simulink model "Inverter_bldc"  (R2020b)
settings: Solver=VariableStepAuto  StartTime=0.0  StopTime=10.0  RelTol=1e-3
undefined symbols (not defined in the file or in its folder): inv
settings Model: Creator=giuli  LastModifiedBy=giuli

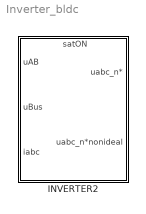
== system Inverter_bldc ==
  INVERTER2 : Subsystem
      settings: PortSchema="{\"entries\":[{\"content\":{\"sides\":[{\"content\":{\"connectorIds\":[\"In1\",\"In2\",\"In3\"]},\"type\":\"ConnectorPlacement.EquallySpacedRectSide\",\"uuid\":\"79c77d12-022f-42ce-98d0-f3ead9d04a95\"},{\"content\":{\"connectorIds\":[\"Out1\",\"Out2\"],\"side\":\"RIGHT\"},\"type\":\"ConnectorPlacement.EquallySpacedRectSide\",\"uuid\":\"afd498dc-a72a-45ee-96a4-44488bf591ce\"},{\"content\":{\"connectorIds\":[\"Out3\"],\"side\":\"TOP\"},\"type\":\"ConnectorPlacement.EquallySpacedRectSide\",\"uuid\":\"f8f8ad46-d0da-4286-941c-855cc15ed51d\"}]},\"type\":\"ConnectorPlacement.EquallySpacedConnector\",\"uuid\":\"436ef73d-4718-409e-82fb-57ff2ccd93cf\"}],\"packageUris\":[\"http://schema.mathworks.com/mf0/Connector/R2020b\"],\"version\":\"1.0\"}"

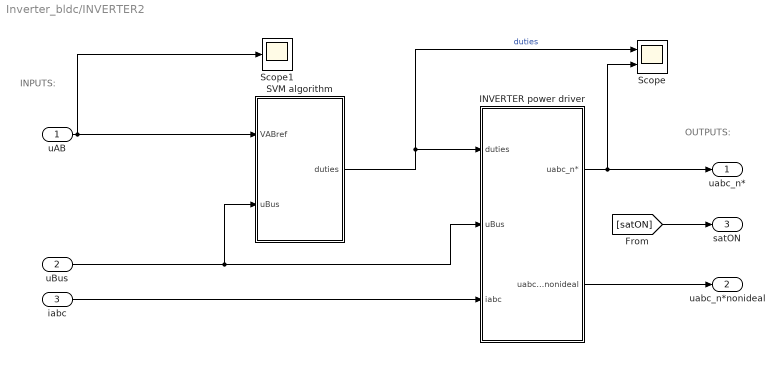
== system Inverter_bldc/INVERTER2 ==
  note: OUTPUTS:
  note: INPUTS:
  uAB : Inport
  uBus : Inport  Port=2
  iabc : Inport  Port=3
  INVERTER power driver : Subsystem
  SVM algorithm : Subsystem
  Scope : Scope  NumInputPorts=2
  Scope1 : Scope
  uabc_n* : Outport
  uabc_n*nonideal : Outport  Port=2
  satON : Outport  Port=3
  wires:
  INVERTER power driver/2(uabc_n*nonideal) -> uabc_n*nonideal/1
  iabc/1 -> INVERTER power driver/3(iabc)
  SVM algorithm/1(duties) -> Scope/1, INVERTER power driver/1(duties)  "duties"
  [satON] -> satON/1
  uBus/1 -> INVERTER power driver/2(uBus), SVM algorithm/2(uBus)
  uAB/1 -> Scope1/1, SVM algorithm/1(VABref)
  INVERTER power driver/1(uabc_n*) -> Scope/2, uabc_n*/1

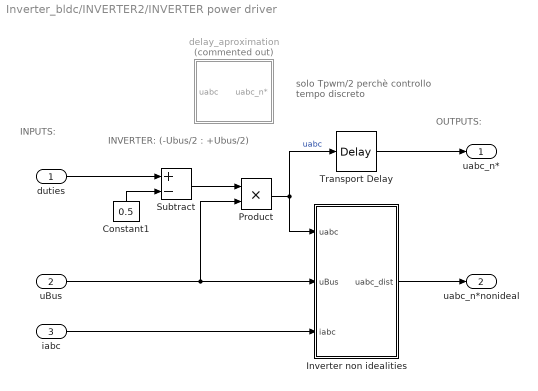
== system Inverter_bldc/INVERTER2/INVERTER power driver ==
  note: INVERTER:
      | (-Ubus/2  :  +Ubus/2)
  note: INPUTS:
  note: OUTPUTS:
  note: solo Tpwm/2 perchè
      | controllo tempo discreto
  duties : Inport
  uBus : Inport  Port=2
  iabc : Inport  Port=3
  Constant1 : Constant  Value=0.5
  Inverter non idealities : Subsystem
  Product : Product
  Subtract : Sum  Inputs=+-
  Transport Delay : TransportDelay  DelayTime=inv.Tpwm/2
  delay_aproximation : Subsystem  Commented=on
  uabc_n* : Outport
  uabc_n*nonideal : Outport  Port=2
  wires:
  iabc/1 -> Inverter non idealities/3(iabc)
  duties/1 -> Subtract/1
  Inverter non idealities/1(uabc_dist) -> uabc_n*nonideal/1
  Constant1/1 -> Subtract/2
  uBus/1 -> Inverter non idealities/2(uBus), Product/2
  Product/1 -> Inverter non idealities/1(uabc), Transport Delay/1  "uabc"
  Subtract/1 -> Product/1
  Transport Delay/1 -> uabc_n*/1

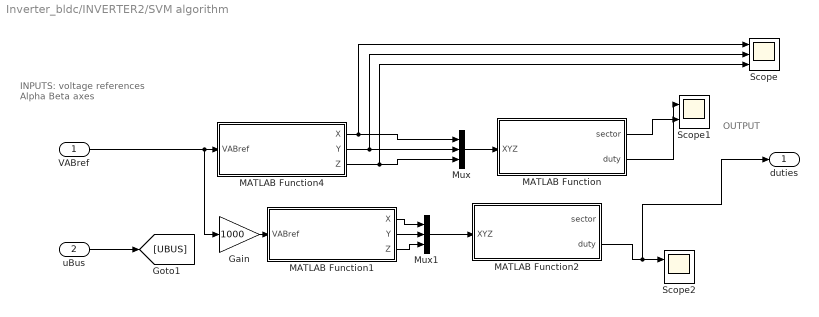
== system Inverter_bldc/INVERTER2/SVM algorithm ==
  note: INPUTS:
      | voltage references
      | Alpha Beta axes
  note: OUTPUT
  VABref : Inport  PortDimensions=2
  uBus : Inport  Port=2  PortDimensions=1
  Gain : Gain  Gain=1000
  MATLAB Function : MATLAB Function  TreatAsAtomicUnit=on  SystemSampleTime=inv.Ts
  MATLAB Function1 : MATLAB Function  TreatAsAtomicUnit=on  SystemSampleTime=inv.Ts
  MATLAB Function2 : MATLAB Function  TreatAsAtomicUnit=on  SystemSampleTime=inv.Ts
  MATLAB Function4 : MATLAB Function  TreatAsAtomicUnit=on  SystemSampleTime=inv.Ts
  Mux : Mux  Inputs=3
  Mux1 : Mux  Inputs=3
  Scope : Scope  NumInputPorts=3
  Scope1 : Scope  NumInputPorts=2
  Scope2 : Scope  NumInputPorts=2
  duties : Outport  PortDimensions=3
  wires:
  Mux/1 -> MATLAB Function/1(XYZ)
  MATLAB Function4/3(Z) -> Scope/3, Mux/3
  MATLAB Function4/2(Y) -> Scope/2, Mux/2
  MATLAB Function4/1(X) -> Scope/1, Mux/1
  MATLAB Function/2(duty) -> Scope1/1
  uBus/1 -> [UBUS]
  VABref/1 -> Gain/1, MATLAB Function4/1(VABref)
  MATLAB Function/1(sector) -> Scope1/2
  MATLAB Function1/3(Z) -> Mux1/3
  MATLAB Function1/2(Y) -> Mux1/2
  MATLAB Function1/1(X) -> Mux1/1
  Gain/1 -> MATLAB Function1/1(VABref)
  Mux1/1 -> MATLAB Function2/1(XYZ)
  MATLAB Function2/2(duty) -> duties/1, Scope2/1

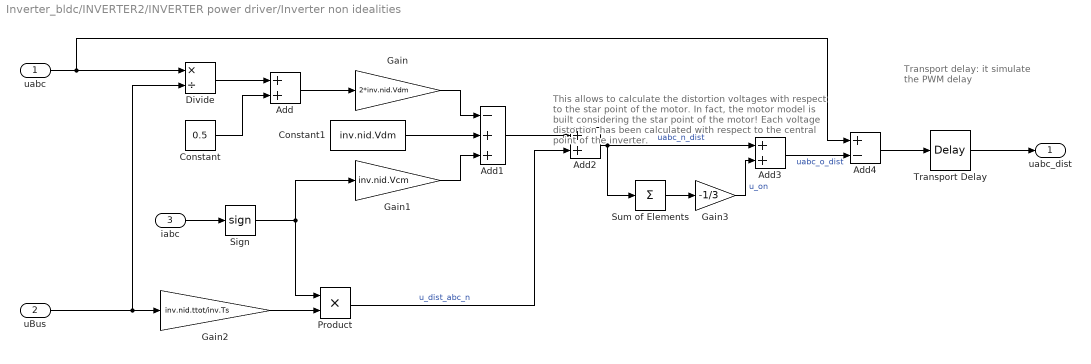
== system Inverter_bldc/INVERTER2/INVERTER power driver/Inverter non idealities ==
  note: This allows to calculate the distortion voltages
      | with respect to the star point of the motor.
      | In fact, the motor model is built considering the
      | star point of the motor! Each voltage distortion
      | has been calculated with respect to the central
      | point of the inverter.
  note: Transport delay: it
      | simulate the PWM
      | delay
  uabc : Inport  PortDimensions=3
  uBus : Inport  Port=2  PortDimensions=1
  iabc : Inport  Port=3  PortDimensions=3
  Add : Sum
  Add1 : Sum  Inputs=-++
  Add2 : Sum
  Add3 : Sum
  Add4 : Sum  Inputs=+-
  Constant : Constant  Value=0.5
  Constant1 : Constant  Value=inv.nid.Vdm
  Divide : Product  Inputs=*/
  Gain : Gain  Gain=2*inv.nid.Vdm
  Gain1 : Gain  Gain=inv.nid.Vcm
  Gain2 : Gain  Gain=inv.nid.ttot/inv.Ts
  Gain3 : Gain  Gain=-1/3
  Product : Product
  Sign : Signum
  Sum of Elements : Sum  Inputs=+
  Transport Delay : TransportDelay  DelayTime=inv.Tpwm/2
  uabc_dist : Outport  PortDimensions=3
  wires:
  Transport Delay/1 -> uabc_dist/1
  Add4/1 -> Transport Delay/1
  Add3/1 -> Add4/2  "uabc_o_dist"
  Gain3/1 -> Add3/2  "u_on"
  Sum of Elements/1 -> Gain3/1
  Add2/1 -> Add3/1, Sum of Elements/1  "uabc_n_dist"
  Product/1 -> Add2/2  "u_dist_abc_n"
  Add1/1 -> Add2/1
  Sign/1 -> Product/1, Gain1/1
  iabc/1 -> Sign/1
  Gain2/1 -> Product/2
  Gain1/1 -> Add1/3
  Constant1/1 -> Add1/2
  Gain/1 -> Add1/1
  Add/1 -> Gain/1
  Divide/1 -> Add/1
  uBus/1 -> Gain2/1, Divide/2
  uabc/1 -> Divide/1, Add4/1
  Constant/1 -> Add/2

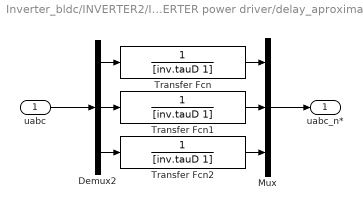
== system Inverter_bldc/INVERTER2/INVERTER power driver/delay_aproximation ==
  uabc : Inport
  Demux2 : Demux  Outputs=3
  Mux : Mux  Inputs=3
  Transfer Fcn : TransferFcn  Denominator=[inv.tauD 1]
  Transfer Fcn1 : TransferFcn  Denominator=[inv.tauD 1]
  Transfer Fcn2 : TransferFcn  Denominator=[inv.tauD 1]
  uabc_n* : Outport
  wires:
  Mux/1 -> uabc_n*/1
  uabc/1 -> Demux2/1
  Demux2/2 -> Transfer Fcn1/1
  Demux2/1 -> Transfer Fcn/1
  Transfer Fcn1/1 -> Mux/2
  Transfer Fcn2/1 -> Mux/3
  Transfer Fcn/1 -> Mux/1
  Demux2/3 -> Transfer Fcn2/1

== matlab function Inverter_bldc/INVERTER2/SVM algorithm/MATLAB Function1 ==
  data: VABref input; X output; Y output; Z output
function [X,Y,Z] = AB2XYZ(VABref)
% this function find the sector in the SVM where uABref is

PWM_period = 5250;
Valpha = VABref(1);
Vbeta = VABref(2);

Ualpha = Valpha * sqrt(3) * PWM_period * 2;
Ubeta = -(Vbeta * PWM_period)* 2;

X = Ubeta;
Y = (Ubeta + Ualpha)/2;
Z = (Ubeta - Ualpha) / 2;
end

== matlab function Inverter_bldc/INVERTER2/SVM algorithm/MATLAB Function2 ==
  data: XYZ input; sector output; duty output
function [sector,duty] = sector_identifier(XYZ)
% this function find the sector in the SVM where uABref is
PWMperiod = 5250;

X = XYZ(1);
Y = XYZ(2);
Z = XYZ(3);

TimePhA = 0;
TimePhB = 0; 
TimePhC = 0;

if(Y < 0) 
    if(Z < 0) 
        sector = 5;
        TimePhA = (PWMperiod/4) + (Y - Z)/262144;
        TimePhB = TimePhA + Z/131072;
        TimePhC = TimePhA - Y/131072;
    else
        if( X <= 0)
            sector = 4;
            TimePhA = (PWMperiod/4) + (X - Z)/262144;
            TimePhB = TimePhA + Z/131072;
            TimePhC = TimePhB - X/131072;
        else
            sector = 3;
            TimePhA = (PWMperiod/4) + (Y - X) /262144;
            TimePhC = TimePhA - Y/131072;
            TimePhB = TimePhC + X/131072;
        end
    end
else
    if(Z>=0)
        sector = 2;
        TimePhA = (PWMperiod/4) + (Y - Z)/262144;
        TimePhB = TimePhA + Z/131072;
        TimePhC = TimePhA - Y/131072;
    else
        if (X<=0)
            sector = 6;
            TimePhA = (PWMperiod/4) + (Y - X) /262144;
            TimePhC = TimePhA - Y/131072;
            TimePhB = TimePhC + X/131072;
        else
            sector = 1;
            TimePhA = (PWMperiod/4) + (X - Z)/262144;
            TimePhB = TimePhA + Z/131072;
            TimePhC = TimePhB - X/131072;
        end
    end
end

duty = [2*TimePhA/5250, 2*TimePhB/5250, 2*TimePhC/5250];
end

== matlab function Inverter_bldc/INVERTER2/SVM algorithm/MATLAB Function ==
  data: XYZ input; sector output; duty output
function [sector,duty] = sector_identifier(XYZ)
% this function find the sector in the SVM where uABref is
PWMperiod = 1/16000;

X = XYZ(1);
Y = XYZ(2);
Z = XYZ(3);

TimePhA = 0;
TimePhB = 0; 
TimePhC = 0;

if(Y < 0) 
    if(Z < 0) 
        sector = 5;
        TimePhA = (PWMperiod/2) + (Y - Z)/2;
        TimePhB = TimePhA + Z;
        TimePhC = TimePhA - Y;
    else
        if( X <= 0)
            sector = 4
            TimePhA = (PWMperiod/2) + (X - Z)/2;
            TimePhB = TimePhA + Z;
            TimePhC = TimePhB - X;
        else
            sector = 3;
            TimePhA = (PWMperiod/2) + (Y - X) /2;
            TimePhC = TimePhA - Y;
            TimePhB = TimePhC + X;
        end
    end
else
    if(Z>=0)
        sector = 2;
        TimePhA = (PWMperiod/2) + (Y - Z)/2;
        TimePhB = TimePhA + Z;
        TimePhC = TimePhA - Y;
    else
        if (X<=0)
            sector = 6;
            TimePhA = (PWMperiod/2) + (Y - X) /2;
            TimePhC = TimePhA - Y;
            TimePhB = TimePhC + X;
        else
            sector = 1;
            TimePhA = (PWMperiod/2) + (X - Z)/2;
            TimePhB = TimePhA + Z;
            TimePhC = TimePhB - X;
        end
    end
end

duty = [TimePhA*16000, TimePhB*16000, TimePhC*16000];
end

== matlab function Inverter_bldc/INVERTER2/SVM algorithm/MATLAB Function4 ==
  data: VABref input; X output; Y output; Z output
function [X,Y,Z] = AB2XYZ(VABref)
% this function find the sector in the SVM where uABref is

PWM_period = 1/16000;
Valpha = VABref(1);
Vbeta = VABref(2);

Ualpha = Valpha * sqrt(3) * PWM_period;
Ubeta = -(Vbeta * PWM_period);

X = Ubeta;
Y = (Ubeta + Ualpha)/2;
Z = (Ubeta - Ualpha) / 2;
end
